simulink model "model_with_phases"  (R2018b)
settings: Solver=VariableStepAuto  StartTime=0.0  StopTime=1  RelTol=1e-3
StopFcn:
  | % fault = 0
  | % %
  | % %
  | % %
  | % %
  | % location = 0
  | % %
  | % %
  | % %
  | % %
  | % %
  | % simout(:,13) = fault;
  | % simout(:,14) = location;
  | % data = xlsread('E:\Project\Simulation\Second\Pavan\samples');
  | % data = [data;simout];
  | % xlswrite('E:\Project\Simulation\Second\Pavan\samples',data);
libraries: powerlib x7, powerlib_meascontrol x2
settings Model: Creator=Edagotti Pavankumar  LastModifiedBy=Edagotti Pavankumar
settings SolverCC: ZeroCrossAlgorithm=Adaptive
settings DebuggingCC: IgnoredZcDiagnostic=none

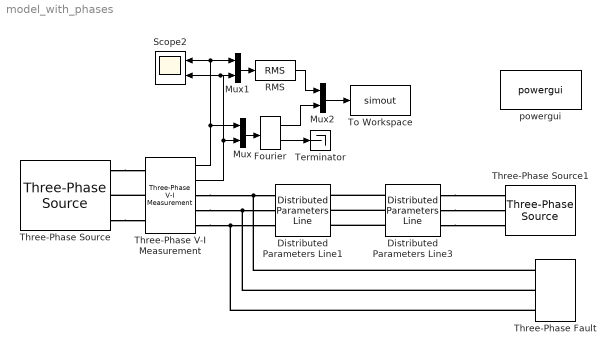
== system model_with_phases ==
  Distributed Parameters Line1 : powerlib/Elements/Distributed Parameters Line  Phases=3  Frequency=50  Resistance=[0.0238 0.3885]  Inductance=[0.0009509508 0.0032508989]  Capacitance=[12.74e-9 7.751e-9]  Length=150  x1=[5.2467676512082e-10 256108.67672753 256108.67672753;314.159265358979 314.159265358979 314.159265358979;2.96054182356813 -0.00741483916072944 -1.57821116595563]  x2=[6.90190834915922e-10 257848.336299754 257848.336299753;314.159265358979 314.159265358979 314.159265358979;3.07452472425731 -0.0331494469154226 -1.60394577371032]  x3=[2.14831057035012e-12 794.188322051418 794.188322051416;314.159265358979 314.159265358979 314.159265358979;2.34502479910533 -0.16519776826205 -1.73599409505695]  x4=[7.67072734039183e-13 1077.49327845534 1077.49327845534;314.159265358979 314.159265358979 314.159265358979;-2.20758631909625 -0.056484771500938 -1.62728109829584]  x5=0.000752959919858122  V1=[5.247e-10 2.561e+05 2.561e+05;314.2 314.2 314.2;2.961 -0.007415 -1.578]  V2=[6.902e-10 2.578e+05 2.578e+05;314.2 314.2 314.2;3.075 -0.03315 -1.604]  I1=[2.148e-12 794.2 794.2;314.2 314.2 314.2;2.345 -0.1652 -1.736]  I2=[7.671e-13 1077 1077;314.2 314.2 314.2;-2.208 -0.05648 -1.627]  nHarmo=1  Measurements=None
      settings: SourceProductName=Simscape Power Systems
  Distributed Parameters Line3 : powerlib/Elements/Distributed Parameters Line  Phases=3  Frequency=50  Resistance=[0.0238 0.3885]  Inductance=[0.0009509508 0.0032508989]  Capacitance=[12.74e-9 7.751e-9]  Length=50  x1=[6.93776961477719e-10 257848.336299754 257848.336299753;314.159265358979 314.159265358979 314.159265358979;-3.05184549240282 0.0761992496837865 -1.49459707711111]  x2=[6.91215973347425e-10 256923.017539917 256923.017539916;314.159265358979 314.159265358979 314.159265358979;3.06274287516733 0.0680934948793638 -1.50270283191554]  x3=[2.82377922060282e-12 797.857371072555 797.857371072553;314.159265358979 314.159265358979 314.159265358979;0.372603313130093 0.107853199475949 -1.46294312731895]  x4=[3.0532719896015e-12 1083.60865135404 1083.60865135404;314.159265358979 314.159265358979 314.159265358979;-2.92261769550343 -0.00163483029360708 -1.57243115708851]  x5=0.000250986639952707  V1=[6.938e-10 2.578e+05 2.578e+05;314.2 314.2 314.2;-3.052 0.0762 -1.495]  V2=[6.912e-10 2.569e+05 2.569e+05;314.2 314.2 314.2;3.063 0.06809 -1.503]  I1=[2.824e-12 797.9 797.9;314.2 314.2 314.2;0.3726 0.1079 -1.463]  I2=[3.053e-12 1084 1084;314.2 314.2 314.2;-2.923 -0.001635 -1.572]  nHarmo=1  Measurements=None
      settings: SourceProductName=Simscape Power Systems
  Fourier : powerlib_meascontrol/Measurements/Fourier  Freq=50  n=1  InInit=[0, 0]  Ts=0
      settings: SourceProductName=Simscape Power Systems
  Mux : Mux  Inputs=2
  Mux1 : Mux  Inputs=2
  Mux2 : Mux  Inputs=2
  RMS : powerlib_meascontrol/Measurements/RMS  TrueRMS=on  Freq=50  RMSInit=0  Ts=0
  Scope2 : Scope  NumInputPorts=2
  Terminator : Terminator
  Three-Phase V-I Measurement : powerlib/Measurements/Three-Phase V-I Measurement  VoltageMeasurement=phase-to-ground  SetLabelV=off  LabelV=Vabc  Vpu=on  VpuLL=off  CurrentMeasurement=yes  SetLabelI=off  LabelI=Iabc  Ipu=on  Pbase=100e6  Vbase=220e3  OutputType=Complex  PhasorSimulation=off  PSBequivalent=0
  Three-Phase Fault : powerlib/Elements/Three-Phase Fault  InitialStates=0  FaultA=on  FaultB=off  FaultC=off  GroundFault=on  SwitchTimes=0.5  External=off  SwitchStatus=NaN  FaultResistance=0.001  GroundResistance=0.001  SnubberResistance=1e6  SnubberCapacitance=inf  Measurements=None
  Three-Phase Source : powerlib/Electrical Sources/Three-Phase Source  InternalConnection=Yg  VoltagePhases=off  Voltage=220e3  PhaseAngle=0  Voltage_phases=[25e3 25e3 25e3]/sqrt(3)  PhaseAngles_phases=[0 -120 +120]  Frequency=50  NonIdealSource=on  SpecifyImpedance=on  Resistance=0.8929  Inductance=16.58e-3  ShortCircuitLevel=100e6  BaseVoltage=220e3  XRratio=7  BusType=swing  Pref=10e3  Qref=0  Prefabc=[10e3, 10e3, 10e3]  Qrefabc=[0, 0, 0]  Qmin=-inf  Qmax=inf
  Three-Phase Source1 : powerlib/Electrical Sources/Three-Phase Source  InternalConnection=Yg  VoltagePhases=off  Voltage=220e3  PhaseAngle=-40  Voltage_phases=[25e3 25e3 25e3]/sqrt(3)  PhaseAngles_phases=[0 -120 +120]  Frequency=50  NonIdealSource=on  SpecifyImpedance=on  Resistance=0.8929  Inductance=16.58e-3  ShortCircuitLevel=100e6  BaseVoltage=220e3  XRratio=7  BusType=PV  Pref=inf  Qref=0  Prefabc=[10e3, 10e3, 10e3]  Qrefabc=[0, 0, 0]  Qmin=-inf  Qmax=inf
  To Workspace : ToWorkspace  VariableName=simout  SampleTime=-1
      settings: MaxDataPoints=200  Save2DSignal=2-D array (concatenate along first dimension)
  powergui : powerlib/powergui  Priority=1  SimulationMode=Continuous  SampleTime=50e-10  frequency=60  Iterations=50  frequencyindice=50  Pbase=100e6  ErrMax=1e-4  UnitsV=kV  UnitsW=MW  buscounter=0  FunctionMessages=off  echomessages=off  EnableUseOfTLC=off  CurrentSourceSwitches=off  DisableSnubberDevices=off  DisableRonSwitches=off  DisableVfSwitches=off  DisplayEquations=off  SolverType=Tustin/Backward Euler (TBE)  Interpol=off  ExternalGateDelay=off  methode=off  Ts=100  x0status=blocks  SPID=off  SwTol=0  HookPort=off  RestoreLinks=warning  ResistiveCurrentMeasurement=off  Frange=[0:2:500]  Ylog=off  Xlog=on  ShowGrid=off  save=off  variable=ZData  structure=0  ZoomFFT=off  StartTime=0.0  cycles=1  DisplayStyle=1  fundamental=60  FreqAxis=off  MaxFrequency=1000  frequencyindicesteady=1  RmsSteady=2  display=off
  wires:
  Fourier/1 -> Terminator/1
  Mux/1 -> Fourier/1
  Mux2/1 -> To Workspace/1
  Three-Phase V-I Measurement/2 -> Mux/2, Scope2/2, Mux1/2
  RMS/1 -> Mux2/1
  Three-Phase V-I Measurement/1 -> Mux/1, Mux1/1, Scope2/1
  Mux1/1 -> RMS/1
  Fourier/2 -> Mux2/2
  connections:
  Three-Phase V-I Measurement/RConn2 -- Three-Phase Fault/LConn2 -- Distributed Parameters Line1/LConn2
  Three-Phase V-I Measurement/RConn1 -- Three-Phase Fault/LConn1 -- Distributed Parameters Line1/LConn1
  Three-Phase V-I Measurement/RConn3 -- Three-Phase Fault/LConn3 -- Distributed Parameters Line1/LConn3
  Three-Phase Source/RConn1 -- Three-Phase V-I Measurement/LConn1
  Distributed Parameters Line3/RConn1 -- Three-Phase Source1/RConn1
  Distributed Parameters Line3/LConn2 -- Distributed Parameters Line1/RConn2
  Distributed Parameters Line3/RConn2 -- Three-Phase Source1/RConn2
  Three-Phase Source/RConn3 -- Three-Phase V-I Measurement/LConn3
  Distributed Parameters Line3/LConn3 -- Distributed Parameters Line1/RConn3
  Three-Phase V-I Measurement/LConn2 -- Three-Phase Source/RConn2
  Distributed Parameters Line3/RConn3 -- Three-Phase Source1/RConn3
  Distributed Parameters Line3/LConn1 -- Distributed Parameters Line1/RConn1
